simulink library "myLibrary"  (R2023b)
settings: Solver=VariableStepAuto  StartTime=0.0  StopTime=10.0  RelTol=1e-3
undefined symbols (not defined in the file): Cac_n1, ctrl1, Da, Discrete, dtha, ee_sli_rtmsupport, FA, gcbh, Ha, Ini, init_DCline, init_IPC, init_line, init_load, init_SG, init_shunt, init_TH, init_trafo, init_VSC, initMachineBlocks, Ka, Lf, Llkd_pu, Llkq1_pu, magnitude, NET, P, plots_step, q0, Rac_n1, Radd, Rkd_pu, Rkq1_pu, Rload_add, sim_config, sps_rtmsupport, spsSteamTurbineModel, T_DC_NET, T_global, T_IPC, T_load, T_NET, T_SG, T_shunt, T_STATCOM, T_TH, T_trafo, T_VSC, Ts, tstep, Udiff_a, V1
libraries: spsSeriesRLCBranchLib x105, eeGeneralControl x72, $bdroot x70, spsCurrentMeasurementLib x48, spsParallelRLCBranchLib x39, spsVoltageMeasurementLib x33, spsControlledVoltageSourceLib x27, spsFirstOrderFilterLib x16, dspsigops x6, spsThreePhaseVIMeasurementLib x5, spsPLL3phLib x4, spsThreePhaseBreakerLib x3
(part 4 of 12)

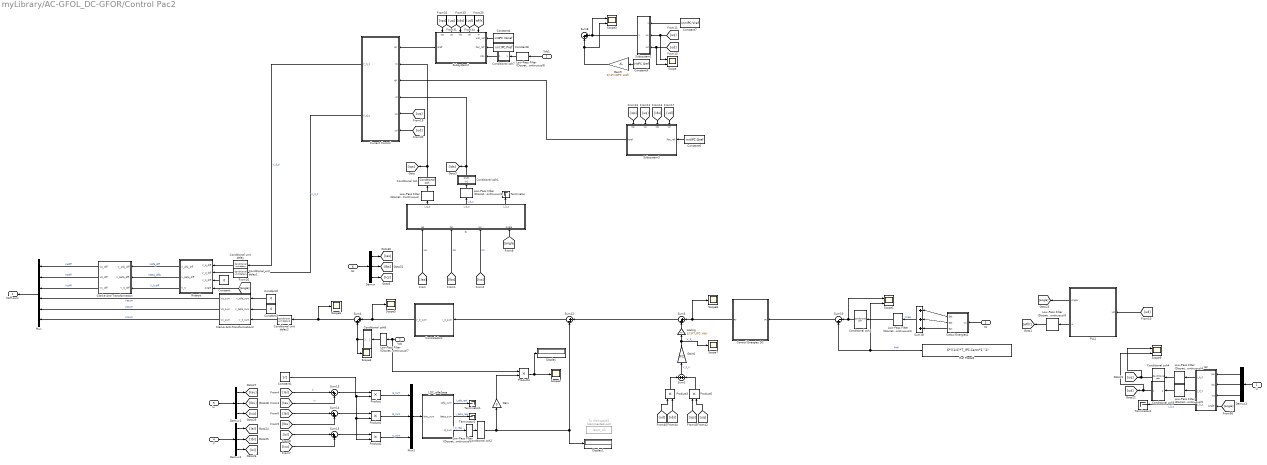
== system myLibrary/AC-GFOL_DC-GFOR/Control Pac2 ==
  U : Inport
  Vdc : Inport  Port=2
  Vs : Inport  Port=3
  Il : Inport  Port=4
  Iu : Inport  Port=5
  Iss : Inport  Port=6
  Calcul Energies2 : Subsystem
  Clarke Anti-Transformation : Subsystem
  Clarke Anti-Transformation2 : Subsystem
  Conditional unit delay : $bdroot/GFOL/Control/Conditional unit delay  SystemSampleTime=-1  VariantActivationTime=update diagram  AllowFlexibleInterface=on  Latency=0  AutoFrameSizeCalculation=off
      link override Constant4: Value=T_IPC.tau_cmd
      link override Unit Delay2: InitialCondition=initIPC.vdiffq  SampleTime=T_IPC.tau_cmd
  Conditional unit delay1 : $bdroot/AC-GFOL_DC-GFOL/Control Pac2/Conditional unit delay1  SystemSampleTime=-1  VariantActivationTime=update diagram  AllowFlexibleInterface=on  Latency=0  AutoFrameSizeCalculation=off
  Conditional unit delay2 : $bdroot/AC-GFOL_DC-GFOL/Control Pac2/Conditional unit delay2  SystemSampleTime=-1  VariantActivationTime=update diagram  AllowFlexibleInterface=on  Latency=0  AutoFrameSizeCalculation=off
  Conditional zoh{,2..4} (4 alike) : $bdroot/AC-GFOL_DC-GFOL/Control Pac2/Conditional zoh  SystemSampleTime=-1  VariantActivationTime=update diagram  AllowFlexibleInterface=on  Latency=0  AutoFrameSizeCalculation=off
  Conditional zoh1 : Subsystem
  Conditional zoh5 : Subsystem
  Conditional zoh7 : Subsystem
  Conditional zoh8 : Subsystem
  Constant : Constant  Value=0
  Constant1 : Constant  Value=1/2
  Constant2 : Constant  Value=0
  Constant3 : Constant  Value=0
  Constant4 : Constant  Value=initIPC.Vdcref
  Constant6 : Constant  Value=initIPC.Qref
  Constant7 : Constant  Value=initIPC.Vref
  Constant8 : Constant  Value=initIPC.Pref
  Constant9 : Constant  Value=initIPC.Qref
  Control Energies DC : Subsystem
  Controladors : Subsystem
  Current Control : Subsystem
  Demux{,1..3} (4 alike) : Demux  Outputs=3
  Display : Display
  Display1 : Display
  Gain : Gain  Gain=3
  Gain6 : Gain  Gain=3/2
  Gain9 : Gain  Gain=2/(3*initIPC.Vref)
  Is : Subsystem
  Is2 : Subsystem
  Low-Pass Filter (Discrete or Continuous) : eeGeneralControl/Low-Pass Filter (Discrete or Continuous)  K=1  T=T_IPC.delay  B=inf  A=-inf  init_option=Specify as parameter  x0=initIPC.idiffq  Ts=0
  Low-Pass Filter (Discrete or Continuous)1 : eeGeneralControl/Low-Pass Filter (Discrete or Continuous)  K=1  T=T_IPC.delay  B=inf  A=-inf  init_option=Specify as parameter  x0=initIPC.idiffd  Ts=0
  Low-Pass Filter (Discrete or Continuous)3 : eeGeneralControl/Low-Pass Filter (Discrete or Continuous)  K=1  T=T_IPC.delay  B=inf  A=-inf  init_option=Specify as parameter  x0=6*((1/2)*T_IPC.Carm*1^2)  Ts=0
  Low-Pass Filter (Discrete or Continuous)4 : eeGeneralControl/Low-Pass Filter (Discrete or Continuous)  K=1  T=T_IPC.delay  B=inf  A=-inf  init_option=Specify as parameter  x0=initIPC.uq  Ts=0
  Low-Pass Filter (Discrete or Continuous)5 : eeGeneralControl/Low-Pass Filter (Discrete or Continuous)  K=1  T=T_IPC.delay  B=inf  A=-inf  init_option=Specify as parameter  x0=initIPC.ud  Ts=0
  Low-Pass Filter (Discrete or Continuous)6 : eeGeneralControl/Low-Pass Filter (Discrete or Continuous)  K=1  T=T_IPC.delay  B=inf  A=-inf  init_option=Specify as parameter  x0=initIPC.isum0_DC  Ts=0
  Low-Pass Filter (Discrete or Continuous)7 : eeGeneralControl/Low-Pass Filter (Discrete or Continuous)  K=1  T=T_IPC.delay  B=inf  A=-inf  init_option=Specify as parameter  x0=initIPC.Vdc  Ts=0
  Low-Pass Filter (Discrete or Continuous)8 : eeGeneralControl/Low-Pass Filter (Discrete or Continuous)  K=1  T=T_IPC.delay  B=inf  A=-inf  init_option=Specify as parameter  x0=initIPC.Vdc  Ts=0
  Low-Pass Filter (Discrete or Continuous)9 : eeGeneralControl/Low-Pass Filter (Discrete or Continuous)  K=1  T=T_IPC.tw  B=inf  A=-inf  init_option=Specify as parameter  x0=2*pi*T_IPC.fb  Ts=0
  Mux : Mux  Inputs=6
  Mux2 : Mux  Inputs=3
  PLL1 : Subsystem
  Product{,1..5} (6 alike) : Product
  Ref Ptotal2 : Constant  Value=6*((1/2)*T_IPC.Carm*1^2)
  Rotació : Subsystem
  Scope{,1,3,9} (4 alike) : Scope  NumInputPorts=2
  Scope{2,4..8} (6 alike) : Scope
  Subsystem1 : Subsystem
      settings: PortSchema="{\"entries\":[{\"content\":{\"sides\":[{\"content\":{\"connectorIds\":[\"Out1\"]},\"type\":\"ConnectorPlacement.EquallySpacedRectSide\",\"uuid\":\"effe47ce-951a-4fb1-8fc1-e963775b8c82\"},{\"content\":{\"connectorIds\":[\"In1\",\"In2\",\"In3\"],\"side\":\"RIGHT\"},\"type\":\"ConnectorPlacement.EquallySpacedRectSide\",\"uuid\":\"a859b59d-6664-4e67-878a-4ecbefd8f8f0\"},{\"content\":{\"connectorIds\":[],\"side\":\"TOP\"},\"type\":\"ConnectorPlacement.EquallySpacedRectSide\",\"uuid\":\"0b762440-c8d9-40a7-a5db-13c46bc0406e\"}]},\"type\":\"ConnectorPlacement.EquallySpacedConnector\",\"uuid\":\"dbc4fef9-6b40-4568-97c6-19f27935f422\"}],\"packageUris\":[\"http://schema.mathworks.com/mf0/Connector/R2020b\"],\"version\":\"1.0\"}"
  Subsystem2 : Subsystem
      settings: PortSchema="{\"entries\":[{\"content\":{\"sides\":[{\"content\":{\"connectorIds\":[\"Out1\"]},\"type\":\"ConnectorPlacement.EquallySpacedRectSide\",\"uuid\":\"dea8424c-00e8-4bd8-a696-176e9d81b4b0\"},{\"content\":{\"connectorIds\":[\"In6\",\"In7\",\"In8\"],\"side\":\"RIGHT\"},\"type\":\"ConnectorPlacement.EquallySpacedRectSide\",\"uuid\":\"15b830a2-0897-480b-96a6-ff349e082a47\"},{\"content\":{\"connectorIds\":[\"In1\",\"In2\",\"In3\",\"In4\",\"In5\"],\"side\":\"TOP\"},\"type\":\"ConnectorPlacement.EquallySpacedRectSide\",\"uuid\":\"07916eec-e3fd-4ba3-9129-5b3a9aa06051\"}]},\"type\":\"ConnectorPlacement.EquallySpacedConnector\",\"uuid\":\"22000632-3c2a-414c-a4d7-471046f1c1a1\"}],\"packageUris\":[\"http://schema.mathworks.com/mf0/Connector/R2020b\"],\"version\":\"1.0\"}"
  Subsystem3 : Subsystem  AncestorBlock=myLibrary/AC-GFOL_DC-GFOR/Control Pac2/Subsystem2
      settings: PortSchema="{\"entries\":[{\"content\":{\"sides\":[{\"content\":{\"connectorIds\":[\"Out1\"]},\"type\":\"ConnectorPlacement.EquallySpacedRectSide\",\"uuid\":\"dea8424c-00e8-4bd8-a696-176e9d81b4b0\"},{\"content\":{\"connectorIds\":[\"In5\"],\"side\":\"RIGHT\"},\"type\":\"ConnectorPlacement.EquallySpacedRectSide\",\"uuid\":\"15b830a2-0897-480b-96a6-ff349e082a47\"},{\"content\":{\"connectorIds\":[\"In1\",\"In2\",\"In3\",\"In4\"],\"side\":\"TOP\"},\"type\":\"ConnectorPlacement.EquallySpacedRectSide\",\"uuid\":\"07916eec-e3fd-4ba3-9129-5b3a9aa06051\"}]},\"type\":\"ConnectorPlacement.EquallySpacedConnector\",\"uuid\":\"22000632-3c2a-414c-a4d7-471046f1c1a1\"}],\"packageUris\":[\"http://schema.mathworks.com/mf0/Connector/R2020b\"],\"version\":\"1.0\"}"
  Sum1 : Sum
  Sum12 : Sum  Inputs=|+-
  Sum{3..4,8,13..15} (6 alike) : Sum  Inputs=|++
  Sum18 : Sum  Inputs=|+++
  Sum19 : Sum  Inputs=|-+
  Terminator{,1..2,4} (4 alike) : Terminator
  To Workspace2 : ToWorkspace  Commented=on  VariableName=isum_n1  SampleTime=plots_step
  Vdc1 : InportShadow  Port=2
  l_DC_alfa/beta : Subsystem
  scaling : Gain  Gain=1/(3*T_IPC.Vdc)
  Vdiff-sum : Outport
  wires:
  Low-Pass Filter (Discrete or Continuous)9/1 -> [wfilt]
  PLL1/2(w) -> Low-Pass Filter (Discrete or Continuous)9/1
  Is/3(I_0_s) -> Terminator/1
  Low-Pass Filter (Discrete or Continuous)7/1 -> Conditional zoh8/1(In1)
  Low-Pass Filter (Discrete or Continuous)3/1 -> Conditional zoh3/1
  Low-Pass Filter (Discrete or Continuous)4/1 -> Conditional zoh4/1
  Low-Pass Filter (Discrete or Continuous)5/1 -> Conditional zoh5/1(In1)
  Low-Pass Filter (Discrete or Continuous)1/1 -> Conditional zoh1/1(In1)
  Low-Pass Filter (Discrete or Continuous)/1 -> Conditional zoh/1
  Ref Ptotal2/1 -> Scope1/2, Sum19/2  "Pref"
  Calcul Energies2/1(Eat) -> Sum18/1
  Constant2/1 -> Clarke Anti-Transformation2/1(V_alfa_sum)
  Constant3/1 -> Clarke Anti-Transformation2/2(V_beta_sum)
  Mux/1 -> Vdiff-sum/1
  Clarke Anti-Transformation2/1(Va_sum) -> Mux/4  "Vasum"
  Clarke Anti-Transformation2/2(Vb_sum) -> Mux/5  "Vbsum"
  Clarke Anti-Transformation/3(Vc_diff) -> Mux/3  "Vcdiff"
  Clarke Anti-Transformation/2(Vb_diff) -> Mux/2  "Vbdiff"
  Clarke Anti-Transformation/1(Va_diff) -> Mux/1  "Vadiff"
  Rotació/1(V_alfa_diff) -> Clarke Anti-Transformation/1(V_alfa_diff)  "Valfa_diff"
  Rotació/3(V_0) -> Clarke Anti-Transformation/3(V_0_diff)  "V_0_diff"
  [Ias] -> Is/1(Ias)  "Ias"
  [Ics] -> Is/3(Ics)  "Ics"
  [Ibs] -> Is/2(Ibs)  "Ibs"
  Rotació/2(V_beta_diff) -> Clarke Anti-Transformation/2(V_beta_dfff)  "Vbeta_diffa"
  Mux2/1 -> l_DC_alfa/beta/1(Iabc_sum)
  Product/1 -> Mux2/1  "Ia_sum"
  [Ial] -> Sum13/1  "Il"
  [Iau] -> Sum13/2  "Iu"
  Sum13/1 -> Product/1
  Constant1/1 -> Product2/2, Product1/2, Product/2
  Product1/1 -> Mux2/2  "Ib_sum"
  [Ibl] -> Sum14/1
  [Ibu] -> Sum14/2
  Sum14/1 -> Product1/1
  Product2/1 -> Mux2/3  "Ic_sum"
  [Icl] -> Sum15/1
  [Icu] -> Sum15/2
  Sum15/1 -> Product2/1
  Clarke Anti-Transformation2/3(Vc_sum) -> Mux/6  "Vcsum"
  Iu/1 -> Demux1/1
  Demux2/2 -> [Ibl]
  Demux1/1 -> [Iau]
  Demux1/3 -> [Icu]
  Il/1 -> Demux2/1
  Demux2/3 -> [Icl]
  Demux2/1 -> [Ial]
  Demux1/2 -> [Ibu]
  Demux3/2 -> Is2/2(Ibs)
  [angle] -> Is2/4(Angle)
  PLL1/1(Angle) -> [angle]
  [ud] -> PLL1/1(Ud)
  U/1 -> Demux3/1
  Demux3/3 -> Is2/3(Ics)
  Demux3/1 -> Is2/1(Ias)
  Demux/1 -> [Ias]
  Demux/2 -> [Ibs]
  Demux/3 -> [Ics]
  Iss/1 -> Demux/1
  Vs/1 -> Calcul Energies2/1(Vs)
  Calcul Energies2/3(Ect) -> Sum18/3
  Calcul Energies2/2(Ebt) -> Sum18/2
  [angle] -> Is/4(Angle)
  [angle] -> Rotació/4(Angle)
  Current Control/1(V_q_s) -> Conditional unit delay/1  "V_0_s"
  [uq] -> Current Control/5(uq)
  [ud] -> Current Control/6(ud)
  Controladors/1(V_0_sum) -> Scope5/1, Sum4/1
  Sum12/1 -> Controladors/1(I_0_sum)
  Sum19/1 -> Control Energies DC/1(Pt)
  Constant7/1 -> Subsystem1/1(uref)
  [uq] -> Scope/1, Subsystem1/2(uq)
  [ud] -> Scope/2, Subsystem1/3(ud)
  Sum4/1 -> Scope6/1, Conditional unit delay2/1
  Is2/3(I_0_s) -> Terminator4/1  "I_0_s"
  Subsystem2/1(iqref) -> Current Control/1(Iq*)
  [ud] -> Product3/1
  [uq] -> Product5/2
  Gain6/1 -> Scope7/1, scaling/1  "V_0_"
  Sum1/1 -> Gain6/1  "V_0_s"
  Product5/1 -> Sum1/2
  Control Energies DC/1(Pt') -> Scope8/1, Sum3/1
  [iqs] -> Product5/1
  scaling/1 -> Sum3/2
  Sum3/1 -> Sum12/1
  Product3/1 -> Sum1/1
  [ids] -> Product3/2
  Subsystem1/1(idref) -> Scope3/1, Sum8/1
  Constant9/1 -> Gain9/1
  Gain9/1 -> Scope3/2, Sum8/2
  Current Control/2(V_d_s) -> Conditional unit delay1/1  "V_0_s"
  Constant/1 -> Rotació/3(V_0_diff)
  l_DC_alfa/beta/1(Ialfa_sum) -> Terminator1/1  "I_afa_real"
  l_DC_alfa/beta/2(Ibeta_sum) -> Terminator2/1  "I_beta_real"
  Constant8/1 -> Subsystem2/7(Pac_ref)
  Vdc1/1 -> Low-Pass Filter (Discrete or Continuous)8/1
  Low-Pass Filter (Discrete or Continuous)8/1 -> Conditional zoh7/1(In1)
  Constant4/1 -> Subsystem2/6(Vdc_ref)
  [wfilt] -> Subsystem2/5(w)
  [ud] -> Subsystem2/4(ud)
  [ids] -> Subsystem2/3(ids)
  [uq] -> Subsystem2/2(uq)
  [iqs] -> Subsystem2/1(iqs)
  Gain/1 -> Product4/2
  Product4/1 -> Display/1, Scope2/1
  [uq] -> Subsystem3/2(uq)
  [ud] -> Subsystem3/4(ud)
  [ids] -> Subsystem3/3(ids)
  Constant6/1 -> Subsystem3/5(Pac_ref)
  [iqs] -> Subsystem3/1(iqs)
  Subsystem3/1(iqref) -> Current Control/3(Id*)
  Conditional unit delay1/1 -> Rotació/2(V_d_diff)
  Conditional unit delay/1 -> Rotació/1(V_q_diff)
  Vdc/1 -> Low-Pass Filter (Discrete or Continuous)7/1, Product4/1
  Conditional unit delay2/1 -> Clarke Anti-Transformation2/3(V_0_sum)
  Conditional zoh7/1(Out1) -> Subsystem2/8(Vdc)
  Conditional zoh8/1(Out1) -> Scope4/1, Sum4/2
  l_DC_alfa/beta/3(I0_sum) -> Low-Pass Filter (Discrete or Continuous)6/1  "I_0_real"
  Low-Pass Filter (Discrete or Continuous)6/1 -> Conditional zoh2/1
  Conditional zoh2/1 -> Gain/1, Sum12/2, Display1/1
  Sum18/1 -> Low-Pass Filter (Discrete or Continuous)3/1  "Preal"
  Conditional zoh3/1 -> Scope1/1, Sum19/1
  Is2/1(I_q_s) -> Low-Pass Filter (Discrete or Continuous)4/1
  Is2/2(I_d_s) -> Low-Pass Filter (Discrete or Continuous)5/1
  Conditional zoh5/1(Out1) -> Scope9/2, [ud]
  Conditional zoh4/1 -> Scope9/1, [uq]
  Is/1(I_q_s) -> Low-Pass Filter (Discrete or Continuous)/1
  Conditional zoh/1 -> Current Control/2(Iq), [iqs]
  Is/2(I_d_s) -> Low-Pass Filter (Discrete or Continuous)1/1  "I_d_s"
  Conditional zoh1/1(Out1) -> Current Control/4(Id), [ids]

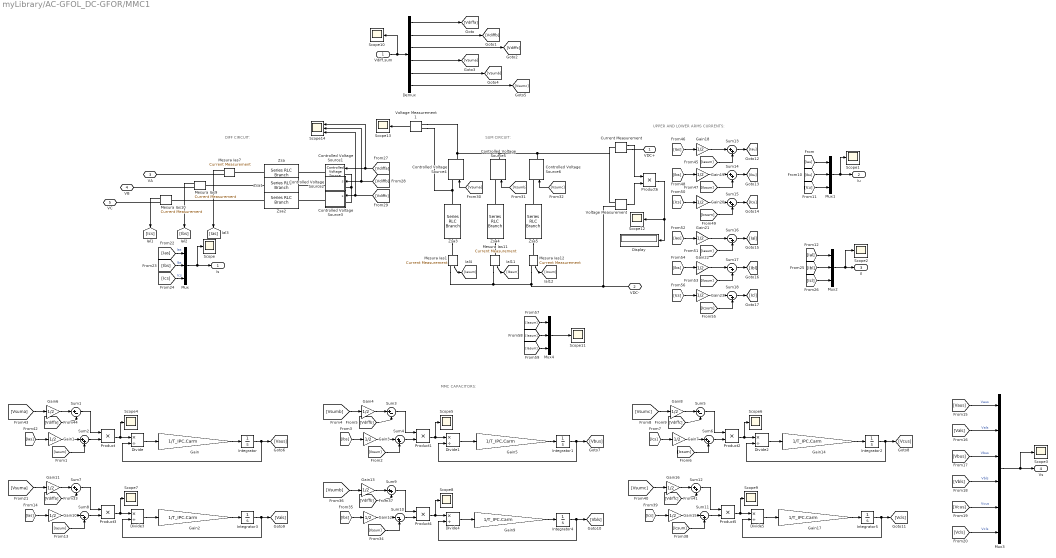
== system myLibrary/AC-GFOL_DC-GFOR/MMC1 ==
  note: DIFF CIRCUIT:
  note: SUM CIRCUIT:
  note: MMC CAPACITORS:
  note: UPPER AND LOWER ARMS CURRENTS:
  Vdiff,sum : Inport
  Controlled Voltage Source1 : spsControlledVoltageSourceLib/Controlled Voltage Source  Initialize=on  Source_Type=AC  Amplitude=initIPC.Udiff_mag  Phase=initIPC.angle_vdiff  Frequency=T_IPC.fb  Measurements=None
  Controlled Voltage Source2 : Subsystem  DialogController=POWERSYS.PowerSysDialog  LoadFcn=sps_rtmsupport('LoadFcn',gcbh);  StartFcn=sps_rtmsupport('StartFcn',gcbh);  StopFcn=sps_rtmsupport('StopFcn',gcbh);  mask(Controlled Voltage Source){Initialize=on, Source_Type=AC, Amplitude=initIPC.Udiff_mag, Phase=initIPC.angle_vdiff-120, Frequency=T_IPC.fb, Measurements=None}
      mask prompts: Source_Type "Source type"; Amplitude "Initial amplitude (V):"; Phase "Initial phase (deg):"; Frequency "Initial frequency (Hz):"
      mask help:
      | Converts the Simulink input signal into an equivalent voltage source. The generated voltage is driven by the input signal of the block.
      |
      | You can initialize your circuit with a specific AC or DC voltage. If you want to start the simulation in steady-state, the block input must be connected to a signal starting as a sinusoidal or DC waveform corresponding to the initial values.
      mask init:
      | powericon('psbloadfunction',gcb,'goto','Initialize');
      | powericon('ControlledSourcesCback',gcb);
      | power_initmask();
      settings: LibrarySourceBlock=spsControlledVoltageSourceLib/Controlled Voltage Source  CopyFcn=sps_rtmsupport('CopyFcn',gcbh); powericon('psbloadfunction',gcb,'goto','UpdateGotoTag');  DeleteFcn=sps_rtmsupport('DeleteFcn',gcbh);  UndoDeleteFcn=sps_rtmsupport('UndoDeleteFcn',gcbh);  ModelCloseFcn=sps_rtmsupport('ModelCloseFcn',gcbh);  PreSaveFcn=sps_rtmsupport('PreSaveFcn',gcbh);  PostSaveFcn=sps_rtmsupport('PostSaveFcn',gcbh);  NameChangeFcn=sps_rtmsupport('NameChangeFcn',gcbh);  PreCopyFcn=sps_rtmsupport('PreCopyFcn',gcbh);  OpenFcn=sps_rtmsupport('OpenFcn',gcbh, [1 2 6]);  CloseFcn=sps_rtmsupport('CloseFcn',gcbh);  PreDeleteFcn=sps_rtmsupport('PreDeleteFcn',gcbh);
      mask Help: helpview(psbhelp);
      mask Callback Initialize: powericon('ControlledSourcesCback',gcb);
      mask TypeOptions Source_Type: AC | DC
      mask Callback Source_Type: powericon('ControlledSourcesCback',gcb);
      mask TypeOptions Measurements: None | Voltage
      mask Display: plot(-50,-35,50,50-15,[0,9,18,24,29,30,29,24,18,9,0,-9,-18,-24,-29,-30,-29,-24,-18,-9,0],[30,29,24,18,9,0,-9,-18,-24,-29,-30,-29,-24,-18,-9,0,9,18,24,29,30],[0,9,18,24,29,30,29,24,18,9,0,-9,-18,-24,-29,-30,-29,-24,-18,-9,0]./-2.4,[1 2 3 4 5 6 7 8 9 10 11 12 13 14 15 16 17 18 19 20 21].*1.5-15);
  Controlled Voltage Source3 : Subsystem  DialogController=POWERSYS.PowerSysDialog  LoadFcn=sps_rtmsupport('LoadFcn',gcbh);  StartFcn=sps_rtmsupport('StartFcn',gcbh);  StopFcn=sps_rtmsupport('StopFcn',gcbh);  mask(Controlled Voltage Source){Initialize=on, Source_Type=AC, Amplitude=initIPC.Udiff_mag, Phase=initIPC.angle_vdiff+120, Frequency=T_IPC.fb, Measurements=None}
      mask prompts: Source_Type "Source type"; Amplitude "Initial amplitude (V):"; Phase "Initial phase (deg):"; Frequency "Initial frequency (Hz):"
      mask help:
      | Converts the Simulink input signal into an equivalent voltage source. The generated voltage is driven by the input signal of the block.
      |
      | You can initialize your circuit with a specific AC or DC voltage. If you want to start the simulation in steady-state, the block input must be connected to a signal starting as a sinusoidal or DC waveform corresponding to the initial values.
      mask init:
      | powericon('psbloadfunction',gcb,'goto','Initialize');
      | powericon('ControlledSourcesCback',gcb);
      | power_initmask();
      settings: LibrarySourceBlock=spsControlledVoltageSourceLib/Controlled Voltage Source  CopyFcn=sps_rtmsupport('CopyFcn',gcbh); powericon('psbloadfunction',gcb,'goto','UpdateGotoTag');  DeleteFcn=sps_rtmsupport('DeleteFcn',gcbh);  UndoDeleteFcn=sps_rtmsupport('UndoDeleteFcn',gcbh);  ModelCloseFcn=sps_rtmsupport('ModelCloseFcn',gcbh);  PreSaveFcn=sps_rtmsupport('PreSaveFcn',gcbh);  PostSaveFcn=sps_rtmsupport('PostSaveFcn',gcbh);  NameChangeFcn=sps_rtmsupport('NameChangeFcn',gcbh);  PreCopyFcn=sps_rtmsupport('PreCopyFcn',gcbh);  OpenFcn=sps_rtmsupport('OpenFcn',gcbh, [1 2 6]);  CloseFcn=sps_rtmsupport('CloseFcn',gcbh);  PreDeleteFcn=sps_rtmsupport('PreDeleteFcn',gcbh);
      mask Help: helpview(psbhelp);
      mask Callback Initialize: powericon('ControlledSourcesCback',gcb);
      mask TypeOptions Source_Type: AC | DC
      mask Callback Source_Type: powericon('ControlledSourcesCback',gcb);
      mask TypeOptions Measurements: None | Voltage
      mask Display: plot(-50,-35,50,50-15,[0,9,18,24,29,30,29,24,18,9,0,-9,-18,-24,-29,-30,-29,-24,-18,-9,0],[30,29,24,18,9,0,-9,-18,-24,-29,-30,-29,-24,-18,-9,0,9,18,24,29,30],[0,9,18,24,29,30,29,24,18,9,0,-9,-18,-24,-29,-30,-29,-24,-18,-9,0]./-2.4,[1 2 3 4 5 6 7 8 9 10 11 12 13 14 15 16 17 18 19 20 21].*1.5-15);
  Controlled Voltage Source4 : spsControlledVoltageSourceLib/Controlled Voltage Source  Initialize=on  Source_Type=DC  Amplitude=initIPC.Usuma  Phase=0  Frequency=0  Measurements=None
  Controlled Voltage Source5 : spsControlledVoltageSourceLib/Controlled Voltage Source  Initialize=on  Source_Type=DC  Amplitude=initIPC.Usumb  Phase=angle(Udiff_a)*180/pi  Frequency=60  Measurements=None
  Controlled Voltage Source6 : spsControlledVoltageSourceLib/Controlled Voltage Source  Initialize=on  Source_Type=DC  Amplitude=initIPC.Usumc  Phase=angle(Udiff_a)*180/pi  Frequency=60  Measurements=None
  Current Measurement : spsCurrentMeasurementLib/Current Measurement  PhasorSimulation=off  OutputType=Complex  PSBequivalent=0
  Demux : Demux  Outputs=6
  Display : Display
  Divide{,1..5} (6 alike) : Product  Inputs=*/
  Gain{,2,5,9,14,17} (6 alike) : Gain  Gain=1/T_IPC.Carm
  Gain{1,3..4,6..8,10..13,15..16,18..23} (18 alike) : Gain  Gain=1/2
  Integrator{,1..5} (6 alike) : Integrator  InitialCondition=1
  Mesura Ias{1,7,9..12} (6 alike) : spsCurrentMeasurementLib/Current Measurement  PhasorSimulation=off  OutputType=Complex  PSBequivalent=0
  Mux{,1..2,4} (4 alike) : Mux  Inputs=3
  Mux3 : Mux  Inputs=6
  Product{,1..6} (7 alike) : Product
  Scope{,1..13} (14 alike) : Scope
  Scope14 : Scope  NumInputPorts=3
  Sum1 : Sum  Inputs=|+-
  Sum{8,10..11,16..18} (6 alike) : Sum  Inputs=|-+
  Sum{2,4,6..7,9,12..15} (9 alike) : Sum  Inputs=|++
  Sum3 : Sum  Inputs=|+-
  Sum5 : Sum  Inputs=|+-
  Voltage Measurement : spsVoltageMeasurementLib/Voltage Measurement  PhasorSimulation=off  OutputType=Complex  PSBequivalent=0
  Voltage Measurement1 : spsVoltageMeasurementLib/Voltage Measurement  PhasorSimulation=off  OutputType=Complex  PSBequivalent=0
  Zsa : spsSeriesRLCBranchLib/Series RLC Branch  LConnTagsString=__new0  RConnTagsString=__new0  BranchType=RL  Resistance=T_IPC.Rc+T_IPC.Ra/2  Inductance=T_IPC.Lc+T_IPC.La/2  SetiL0=on  InitialCurrent=initIPC.Isa  Capacitance=1e-6  Setx0=off  InitialVoltage=0  Measurements=None
  Zsa1 : spsSeriesRLCBranchLib/Series RLC Branch  LConnTagsString=__new0  RConnTagsString=__new0  BranchType=RL  Resistance=T_IPC.Rc+T_IPC.Ra/2  Inductance=T_IPC.Lc+T_IPC.La/2  SetiL0=on  InitialCurrent=initIPC.Isb  Capacitance=1e-6  Setx0=off  InitialVoltage=0  Measurements=None
  Zsa2 : spsSeriesRLCBranchLib/Series RLC Branch  LConnTagsString=__new0  RConnTagsString=__new0  BranchType=RL  Resistance=T_IPC.Rc+T_IPC.Ra/2  Inductance=T_IPC.Lc+T_IPC.La/2  SetiL0=on  InitialCurrent=initIPC.Isc  Capacitance=1e-6  Setx0=off  InitialVoltage=0  Measurements=None
  Zsa3 : spsSeriesRLCBranchLib/Series RLC Branch  LConnTagsString=__new0  RConnTagsString=__new0  BranchType=RL  Resistance=2*T_IPC.Ra  Inductance=2*T_IPC.La  SetiL0=on  InitialCurrent=initIPC.isum0_DC  Capacitance=1e-6  Setx0=off  InitialVoltage=0  Measurements=None
  Zsa4 : spsSeriesRLCBranchLib/Series RLC Branch  LConnTagsString=__new0  RConnTagsString=__new0  BranchType=RL  Resistance=2*T_IPC.Ra  Inductance=2*T_IPC.La  SetiL0=on  InitialCurrent=initIPC.isum0_DC  Capacitance=1e-6  Setx0=off  InitialVoltage=0  Measurements=None
  Zsa5 : spsSeriesRLCBranchLib/Series RLC Branch  LConnTagsString=__new0  RConnTagsString=__new0  BranchType=RL  Resistance=2*T_IPC.Ra  Inductance=2*T_IPC.La  SetiL0=on  InitialCurrent=initIPC.isum0_DC  Capacitance=1e-6  Setx0=off  InitialVoltage=0  Measurements=None
  VDC+ : PMIOPort  Side=Right
  VDC- : PMIOPort  Port=2  Side=Right
  VA : PMIOPort  Port=3  Side=Left
  VB : PMIOPort  Port=4  Side=Left
  VC : PMIOPort  Port=5  Side=Left
  Is : Outport
  Iu : Outport  Port=2
  Il : Outport  Port=3
  Vs : Outport  Port=4
  wires:
  Mux4/1 -> Scope11/1
  [Iasum] -> Mux4/3
  [Iasum] -> Mux4/2
  [Iasum] -> Mux4/1
  Mesura Ias10/1 -> [Ics]
  Mesura Ias7/1 -> [Ias]
  Mesura Ias9/1 -> [Ibs]
  Vdiff,sum/1 -> Demux/1, Scope10/1
  Demux/5 -> [Vsumb]
  Demux/6 -> [Vsumc]
  Demux/1 -> [Vdiffa]
  Demux/3 -> [Vdiffc]
  Demux/2 -> [Vdiffb]
  Demux/4 -> [Vsuma]
  Mux/1 -> Scope/1, Is/1
  [Ics] -> Mux/3  "Ics"
  [Ibs] -> Mux/2  "Ibs"
  [Ias] -> Mux/1  "Ias"
  [Iau] -> Mux1/1
  [Ibu] -> Mux1/2
  [Icu] -> Mux1/3
  Mux1/1 -> Scope1/1, Iu/1
  [Ial] -> Mux2/1
  Mux2/1 -> Scope2/1, Il/1
  [Icl] -> Mux2/3
  [Vaus] -> Mux3/1  "Vaus"
  [Vals] -> Mux3/2  "Vals"
  [Vbus] -> Mux3/3  "Vbus"
  [Vbls] -> Mux3/4  "Vbls"
  [Vcus] -> Mux3/5  "Vcus"
  [Vcls] -> Mux3/6  "Vcls"
  Mux3/1 -> Scope3/1, Vs/1
  Sum2/1 -> Product/2
  Product/1 -> Scope4/1, Divide/1
  Divide/1 -> Gain/1
  Gain/1 -> Integrator/1
  Integrator/1 -> [Vaus], Divide/2
  [Vdiffa] -> Scope14/1, Controlled Voltage Source1/1
  [Vdiffb] -> Scope14/2, Controlled Voltage Source2/1(s)
  Mesura Ias1/1 -> [Iasum]
  Mesura Ias11/1 -> [Ibsum]
  Mesura Ias12/1 -> [Icsum]
  [Vsuma] -> Controlled Voltage Source4/1
  [Vsumb] -> Controlled Voltage Source5/1
  [Vsumc] -> Controlled Voltage Source6/1
  Gain6/1 -> Sum1/1
  [Vdiffa] -> Sum1/2
  [Iasum] -> Sum2/2
  Gain1/1 -> Sum2/1
  [Ias] -> Gain1/1
  [Vsuma] -> Gain6/1
  Sum1/1 -> Product/1
  Sum3/1 -> Product1/1
  [Vsumb] -> Gain4/1
  [Ibs] -> Gain3/1
  Gain3/1 -> Sum4/1
  [Ibsum] -> Sum4/2
  [Vdiffb] -> Sum3/2
  Gain4/1 -> Sum3/1
  Integrator1/1 -> Divide1/2, [Vbus]
  Gain5/1 -> Integrator1/1
  Divide1/1 -> Gain5/1
  Product1/1 -> Divide1/1, Scope5/1
  Sum4/1 -> Product1/2
  Sum6/1 -> Product2/2
  Product2/1 -> Scope6/1, Divide2/1
  Divide2/1 -> Gain14/1
  Gain14/1 -> Integrator2/1
  Integrator2/1 -> [Vcus], Divide2/2
  Gain8/1 -> Sum5/1
  [Vdiffc] -> Sum5/2
  [Icsum] -> Sum6/2
  Gain7/1 -> Sum6/1
  [Ics] -> Gain7/1
  [Vsumc] -> Gain8/1
  Sum5/1 -> Product2/1
  Sum7/1 -> Product3/1
  [Vsuma] -> Gain11/1
  [Ias] -> Gain10/1
  Gain10/1 -> Sum8/1
  [Iasum] -> Sum8/2
  [Vdiffa] -> Sum7/2
  Gain11/1 -> Sum7/1
  Integrator3/1 -> Divide3/2, [Vals]
  Gain2/1 -> Integrator3/1
  Divide3/1 -> Gain2/1
  Product3/1 -> Divide3/1, Scope7/1
  Sum8/1 -> Product3/2
  Sum10/1 -> Product4/2
  Product4/1 -> Scope8/1, Divide4/1
  Divide4/1 -> Gain9/1
  Gain9/1 -> Integrator4/1
  Integrator4/1 -> [Vbls], Divide4/2
  Gain13/1 -> Sum9/1
  [Vdiffb] -> Sum9/2
  [Ibsum] -> Sum10/2
  Gain12/1 -> Sum10/1
  [Ibs] -> Gain12/1
  [Vsumb] -> Gain13/1
  Sum9/1 -> Product4/1
  Sum12/1 -> Product5/1
  [Vsumc] -> Gain16/1
  [Ics] -> Gain15/1
  Gain15/1 -> Sum11/1
  [Icsum] -> Sum11/2
  [Vdiffc] -> Sum12/2
  Gain16/1 -> Sum12/1
  Integrator5/1 -> Divide5/2, [Vcls]
  Gain17/1 -> Integrator5/1
  Divide5/1 -> Gain17/1
  Product5/1 -> Divide5/1, Scope9/1
  Sum11/1 -> Product5/2
  [Ias] -> Gain18/1
  Gain18/1 -> Sum13/1
  [Iasum] -> Sum13/2
  Sum13/1 -> [Iau]
  Sum14/1 -> [Ibu]
  [Ibsum] -> Sum14/2
  Gain19/1 -> Sum14/1
  [Ibs] -> Gain19/1
  [Ics] -> Gain20/1
  Gain20/1 -> Sum15/1
  [Icsum] -> Sum15/2
  Sum15/1 -> [Icu]
  [Iasum] -> Sum16/2
  [Ias] -> Gain21/1
  Gain21/1 -> Sum16/1
  Sum16/1 -> [Ial]
  Sum17/1 -> [Ibl]
  Gain22/1 -> Sum17/1
  [Ibs] -> Gain22/1
  [Ibsum] -> Sum17/2
  [Icsum] -> Sum18/2
  [Ics] -> Gain23/1
  Gain23/1 -> Sum18/1
  Sum18/1 -> [Icl]
  [Ibl] -> Mux2/2
  Current Measurement/1 -> Product6/1
  Voltage Measurement/1 -> Product6/2
  Product6/1 -> Display/1, Scope12/1
  Voltage Measurement1/1 -> Scope13/1
  [Vdiffc] -> Controlled Voltage Source3/1(s), Scope14/3
  connections:
  Zsa5/RConn1 -- Mesura Ias12/LConn1
  Zsa5/LConn1 -- Controlled Voltage Source6/LConn1
  Zsa4/RConn1 -- Mesura Ias11/LConn1
  Zsa4/LConn1 -- Controlled Voltage Source5/LConn1
  Zsa3/RConn1 -- Mesura Ias1/LConn1
  Zsa3/LConn1 -- Voltage Measurement1/LConn2 -- Controlled Voltage Source4/LConn1
  Mesura Ias7/RConn1 -- VA/RConn1
  Mesura Ias9/RConn1 -- VB/RConn1
  Mesura Ias10/RConn1 -- VC/RConn1
  Zsa/RConn1 -- Mesura Ias7/LConn1
  Zsa1/RConn1 -- Mesura Ias9/LConn1
  Zsa2/RConn1 -- Mesura Ias10/LConn1
  Controlled Voltage Source1/RConn1 -- Zsa/LConn1
  Controlled Voltage Source2/RConn1 -- Zsa1/LConn1
  Controlled Voltage Source3/RConn1 -- Zsa2/LConn1
  Controlled Voltage Source1/LConn1 -- Controlled Voltage Source3/LConn1 -- Controlled Voltage Source2/LConn1
  Controlled Voltage Source6/RConn1 -- Current Measurement/LConn1 -- Voltage Measurement/LConn1 -- Controlled Voltage Source5/RConn1 -- Voltage Measurement1/LConn1 -- Controlled Voltage Source4/RConn1
  Mesura Ias1/RConn1 -- Mesura Ias11/RConn1 -- Mesura Ias12/RConn1 -- Voltage Measurement/LConn2 -- VDC-/RConn1
  Current Measurement/RConn1 -- VDC+/RConn1

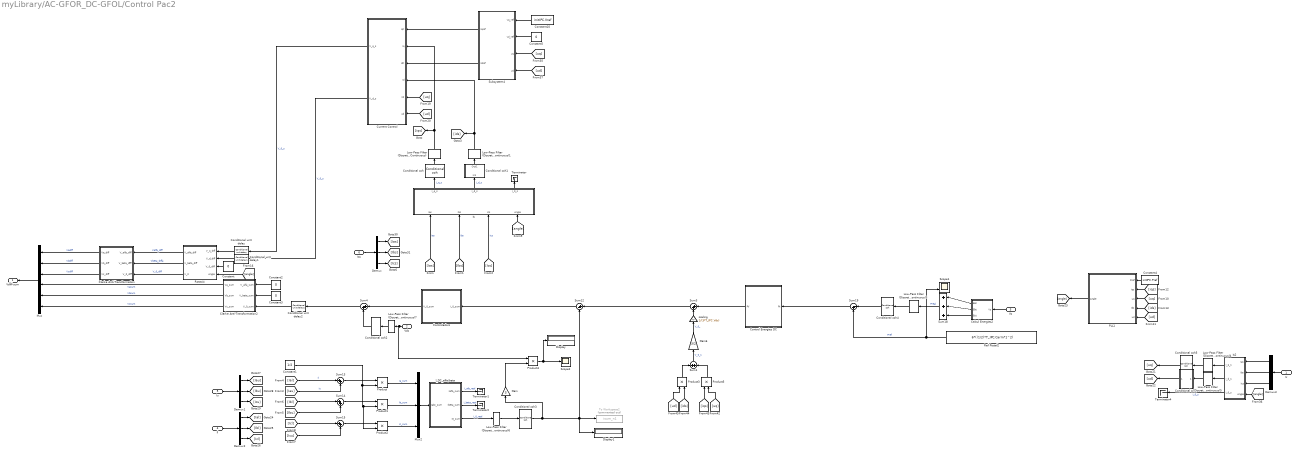
== system myLibrary/AC-GFOR_DC-GFOL/Control Pac2 ==
  U : Inport
  Vdc : Inport  Port=2
  Vs : Inport  Port=3
  Il : Inport  Port=4
  Iu : Inport  Port=5
  Iss : Inport  Port=6
  Calcul Energies2 : Subsystem
  Clarke Anti-Transformation : Subsystem
  Clarke Anti-Transformation2 : Subsystem
  Conditional unit delay : $bdroot/GFOL/Control/Conditional unit delay  SystemSampleTime=-1  VariantActivationTime=update diagram  AllowFlexibleInterface=on  Latency=0  AutoFrameSizeCalculation=off
      link override Constant4: Value=T_IPC.tau_cmd
      link override Unit Delay2: InitialCondition=initIPC.vdiffq  SampleTime=T_IPC.tau_cmd
  Conditional unit delay1 : $bdroot/AC-GFOL_DC-GFOL/Control Pac2/Conditional unit delay1  SystemSampleTime=-1  VariantActivationTime=update diagram  AllowFlexibleInterface=on  Latency=0  AutoFrameSizeCalculation=off
  Conditional unit delay2 : $bdroot/AC-GFOL_DC-GFOL/Control Pac2/Conditional unit delay2  SystemSampleTime=-1  VariantActivationTime=update diagram  AllowFlexibleInterface=on  Latency=0  AutoFrameSizeCalculation=off
  Conditional zoh{,2..5} (5 alike) : $bdroot/AC-GFOL_DC-GFOL/Control Pac2/Conditional zoh  SystemSampleTime=-1  VariantActivationTime=update diagram  AllowFlexibleInterface=on  Latency=0  AutoFrameSizeCalculation=off
  Conditional zoh1 : Subsystem
  Conditional zoh6 : Subsystem
  Constant{,2..3,5} (4 alike) : Constant  Value=0
  Constant1 : Constant  Value=1/2
  Constant10 : Constant  Value=initIPC.Vref
  Constant4 : Constant  Value=initIPC.Pref
  Control Energies DC : Subsystem
  Controladors : Subsystem
  Current Control : Subsystem
  Demux{,1..3} (4 alike) : Demux  Outputs=3
  Display : Display
  Display1 : Display
  Gain : Gain  Gain=3
  Gain6 : Gain  Gain=3/2
  Is : Subsystem
  Is2 : Subsystem
  Low-Pass Filter (Discrete or Continuous) : eeGeneralControl/Low-Pass Filter (Discrete or Continuous)  K=1  T=T_IPC.delay  B=inf  A=-inf  init_option=Specify as parameter  x0=initIPC.idiffq  Ts=0
  Low-Pass Filter (Discrete or Continuous)1 : eeGeneralControl/Low-Pass Filter (Discrete or Continuous)  K=1  T=T_IPC.delay  B=inf  A=-inf  init_option=Specify as parameter  x0=initIPC.idiffd  Ts=0
  Low-Pass Filter (Discrete or Continuous)3 : eeGeneralControl/Low-Pass Filter (Discrete or Continuous)  K=1  T=T_IPC.delay  B=inf  A=-inf  init_option=Specify as parameter  x0=6*((1/2)*T_IPC.Carm*1^2)  Ts=0
  Low-Pass Filter (Discrete or Continuous)4 : eeGeneralControl/Low-Pass Filter (Discrete or Continuous)  K=1  T=T_IPC.delay  B=inf  A=-inf  init_option=Specify as parameter  x0=initIPC.uq  Ts=0
  Low-Pass Filter (Discrete or Continuous)5 : eeGeneralControl/Low-Pass Filter (Discrete or Continuous)  K=1  T=T_IPC.delay  B=inf  A=-inf  init_option=Specify as parameter  x0=initIPC.ud  Ts=0
  Low-Pass Filter (Discrete or Continuous)6 : eeGeneralControl/Low-Pass Filter (Discrete or Continuous)  K=1  T=T_IPC.delay  B=inf  A=-inf  init_option=Specify as parameter  x0=initIPC.isum0_DC  Ts=0
  Low-Pass Filter (Discrete or Continuous)7 : eeGeneralControl/Low-Pass Filter (Discrete or Continuous)  K=1  T=T_IPC.delay  B=inf  A=-inf  init_option=Specify as parameter  x0=initIPC.Vdc  Ts=0
  Mux : Mux  Inputs=6
  Mux2 : Mux  Inputs=3
  PLL1 : Subsystem
  Product{,1..5} (6 alike) : Product
  Ref Ptotal2 : Constant  Value=6*((1/2)*T_IPC.Carm*1^2)
  Rotació : Subsystem
  Scope1 : Scope  NumInputPorts=2
  Scope2 : Scope
  Subsystem4 : Subsystem
  Sum1 : Sum
  Sum12 : Sum  Inputs=|+-
  Sum{3..4,13..15} (5 alike) : Sum  Inputs=|++
  Sum18 : Sum  Inputs=|+++
  Sum19 : Sum  Inputs=|-+
  Terminator{,1..2,4} (4 alike) : Terminator
  To Workspace2 : ToWorkspace  Commented=on  VariableName=isum_n1  SampleTime=plots_step
  l_DC_alfa/beta : Subsystem
  scaling : Gain  Gain=1/(3*T_IPC.Vdc)
  Vdiff-sum : Outport
  wires:
  Product4/1 -> Scope2/1, Display/1
  Gain/1 -> Product4/2
  l_DC_alfa/beta/2(Ibeta_sum) -> Terminator2/1  "I_beta_real"
  l_DC_alfa/beta/1(Ialfa_sum) -> Terminator1/1  "I_afa_real"
  Constant/1 -> Rotació/3(V_0_diff)
  Current Control/2(V_d_s) -> Conditional unit delay1/1  "V_0_s"
  [ids] -> Product3/2
  Product3/1 -> Sum1/1
  Sum3/1 -> Sum12/1
  scaling/1 -> Sum3/2
  [iqs] -> Product5/1
  Control Energies DC/1(Pt') -> Sum3/1
  Product5/1 -> Sum1/2
  Sum1/1 -> Gain6/1  "V_0_s"
  Gain6/1 -> scaling/1  "V_0_"
  [uq] -> Product5/2
  [ud] -> Product3/1
  Subsystem4/1(iqref) -> Current Control/1(Iq*)
  Is2/3(I_0_s) -> Terminator4/1  "I_0_s"
  Sum4/1 -> Conditional unit delay2/1
  Sum19/1 -> Control Energies DC/1(Pt)
  Sum12/1 -> Controladors/1(I_0_sum)
  Controladors/1(V_0_sum) -> Sum4/1
  [ud] -> Current Control/6(ud)
  [uq] -> Current Control/5(uq)
  Current Control/1(V_q_s) -> Conditional unit delay/1  "V_0_s"
  [angle] -> Rotació/4(Angle)
  [angle] -> Is/4(Angle)
  Calcul Energies2/2(Ebt) -> Sum18/2
  Calcul Energies2/3(Ect) -> Sum18/3
  Vs/1 -> Calcul Energies2/1(Vs)
  Iss/1 -> Demux/1
  Demux/3 -> [Ics]
  Demux/2 -> [Ibs]
  Demux/1 -> [Ias]
  Demux3/1 -> Is2/1(Ias)
  Demux3/3 -> Is2/3(Ics)
  U/1 -> Demux3/1
  PLL1/1(Angle) -> [angle]
  [angle] -> Is2/4(Angle)
  Demux3/2 -> Is2/2(Ibs)
  Demux1/2 -> [Ibu]
  Demux2/1 -> [Ial]
  Demux2/3 -> [Icl]
  Il/1 -> Demux2/1
  Demux1/3 -> [Icu]
  Demux1/1 -> [Iau]
  Demux2/2 -> [Ibl]
  Iu/1 -> Demux1/1
  Clarke Anti-Transformation2/3(Vc_sum) -> Mux/6  "Vcsum"
  Sum15/1 -> Product2/1
  [Icu] -> Sum15/2
  [Icl] -> Sum15/1
  Product2/1 -> Mux2/3  "Ic_sum"
  Sum14/1 -> Product1/1
  [Ibu] -> Sum14/2
  [Ibl] -> Sum14/1
  Product1/1 -> Mux2/2  "Ib_sum"
  Constant1/1 -> Product/2, Product1/2, Product2/2
  Sum13/1 -> Product/1
  [Iau] -> Sum13/2  "Iu"
  [Ial] -> Sum13/1  "Il"
  Product/1 -> Mux2/1  "Ia_sum"
  Mux2/1 -> l_DC_alfa/beta/1(Iabc_sum)
  Rotació/2(V_beta_diff) -> Clarke Anti-Transformation/2(V_beta_dfff)  "Vbeta_diffa"
  [Ibs] -> Is/2(Ibs)  "Ibs"
  [Ics] -> Is/3(Ics)  "Ics"
  [Ias] -> Is/1(Ias)  "Ias"
  Rotació/3(V_0) -> Clarke Anti-Transformation/3(V_0_diff)  "V_0_diff"
  Rotació/1(V_alfa_diff) -> Clarke Anti-Transformation/1(V_alfa_diff)  "Valfa_diff"
  Is/1(I_q_s) -> Conditional zoh/1  "I_q_s"
  Is/2(I_d_s) -> Conditional zoh1/1(In1)  "I_d_s"
  Clarke Anti-Transformation/1(Va_diff) -> Mux/1  "Vadiff"
  Clarke Anti-Transformation/2(Vb_diff) -> Mux/2  "Vbdiff"
  Clarke Anti-Transformation/3(Vc_diff) -> Mux/3  "Vcdiff"
  Clarke Anti-Transformation2/2(Vb_sum) -> Mux/5  "Vbsum"
  Clarke Anti-Transformation2/1(Va_sum) -> Mux/4  "Vasum"
  Mux/1 -> Vdiff-sum/1
  Constant3/1 -> Clarke Anti-Transformation2/2(V_beta_sum)
  Constant2/1 -> Clarke Anti-Transformation2/1(V_alfa_sum)
  Calcul Energies2/1(Eat) -> Sum18/1
  Ref Ptotal2/1 -> Sum19/2, Scope1/2  "Pref"
  Low-Pass Filter (Discrete or Continuous)/1 -> [iqs], Current Control/2(Iq)
  Low-Pass Filter (Discrete or Continuous)1/1 -> [ids], Current Control/4(Id)
  Low-Pass Filter (Discrete or Continuous)5/1 -> Conditional zoh6/1(In1)
  Low-Pass Filter (Discrete or Continuous)4/1 -> Conditional zoh5/1
  Low-Pass Filter (Discrete or Continuous)3/1 -> Conditional zoh4/1
  Low-Pass Filter (Discrete or Continuous)7/1 -> Conditional zoh2/1
  Is/3(I_0_s) -> Terminator/1
  Low-Pass Filter (Discrete or Continuous)6/1 -> Conditional zoh3/1
  Constant5/1 -> Subsystem4/2(vd_ref)
  Constant10/1 -> Subsystem4/1(vq_ref)
  [uq] -> Subsystem4/3(vq)
  [ud] -> Subsystem4/4(vd)
  Subsystem4/2(idref) -> Current Control/3(Id*)
  [uq] -> PLL1/3(uq)
  [ud] -> PLL1/5(ud)
  [iqs] -> PLL1/2(iqs)
  [ids] -> PLL1/4(ids)
  Constant4/1 -> PLL1/1(Pref)
  Conditional unit delay1/1 -> Rotació/2(V_d_diff)
  Conditional unit delay/1 -> Rotació/1(V_q_diff)
  Conditional zoh/1 -> Low-Pass Filter (Discrete or Continuous)/1
  Conditional zoh1/1(Out1) -> Low-Pass Filter (Discrete or Continuous)1/1
  Conditional unit delay2/1 -> Clarke Anti-Transformation2/3(V_0_sum)
  Vdc/1 -> Product4/1, Low-Pass Filter (Discrete or Continuous)7/1
  Conditional zoh2/1 -> Sum4/2
  Conditional zoh3/1 -> Sum12/2, To Workspace2/1, Display1/1, Gain/1
  l_DC_alfa/beta/3(I0_sum) -> Low-Pass Filter (Discrete or Continuous)6/1  "I_0_real"
  Is2/1(I_q_s) -> Low-Pass Filter (Discrete or Continuous)4/1
  Is2/2(I_d_s) -> Low-Pass Filter (Discrete or Continuous)5/1
  Conditional zoh6/1(Out1) -> [ud]
  Conditional zoh5/1 -> [uq]
  Sum18/1 -> Low-Pass Filter (Discrete or Continuous)3/1  "Preal"
  Conditional zoh4/1 -> Sum19/1

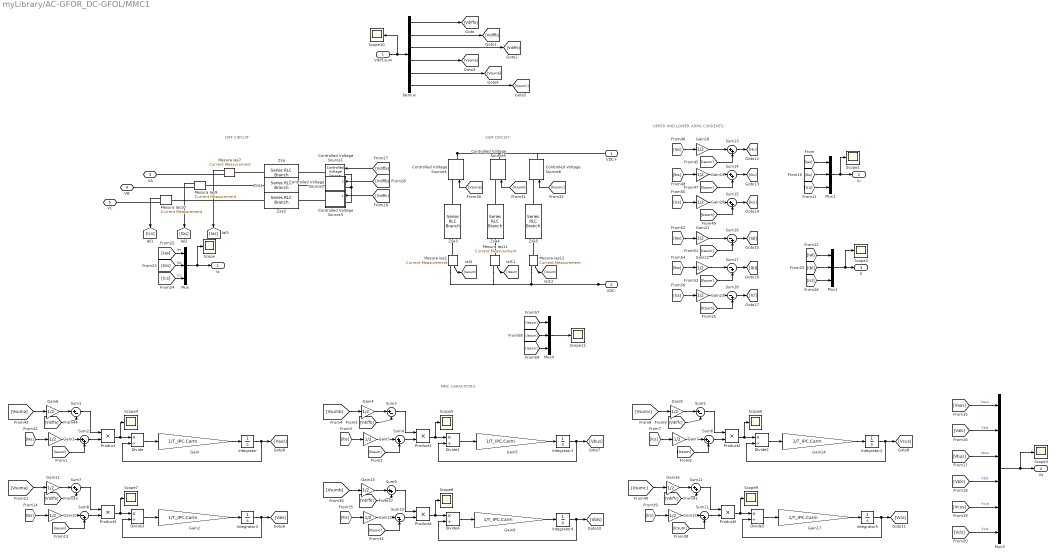
== system myLibrary/AC-GFOR_DC-GFOL/MMC1 ==
  note: UPPER AND LOWER ARMS CURRENTS:
  note: MMC CAPACITORS:
  note: SUM CIRCUIT:
  note: DIFF CIRCUIT:
  Vdiff,sum : Inport
  Controlled Voltage Source1 : spsControlledVoltageSourceLib/Controlled Voltage Source  Initialize=on  Source_Type=AC  Amplitude=initIPC.Udiff_mag  Phase=initIPC.angle_vdiff  Frequency=T_IPC.fb  Measurements=None
  Controlled Voltage Source2 : Subsystem  DialogController=POWERSYS.PowerSysDialog  LoadFcn=sps_rtmsupport('LoadFcn',gcbh);  StartFcn=sps_rtmsupport('StartFcn',gcbh);  StopFcn=sps_rtmsupport('StopFcn',gcbh);  mask(Controlled Voltage Source){Initialize=on, Source_Type=AC, Amplitude=initIPC.Udiff_mag, Phase=initIPC.angle_vdiff-120, Frequency=T_IPC.fb, Measurements=None}
      mask prompts: Source_Type "Source type"; Amplitude "Initial amplitude (V):"; Phase "Initial phase (deg):"; Frequency "Initial frequency (Hz):"
      mask help:
      | Converts the Simulink input signal into an equivalent voltage source. The generated voltage is driven by the input signal of the block.
      |
      | You can initialize your circuit with a specific AC or DC voltage. If you want to start the simulation in steady-state, the block input must be connected to a signal starting as a sinusoidal or DC waveform corresponding to the initial values.
      mask init:
      | powericon('psbloadfunction',gcb,'goto','Initialize');
      | powericon('ControlledSourcesCback',gcb);
      | power_initmask();
      settings: LibrarySourceBlock=spsControlledVoltageSourceLib/Controlled Voltage Source  CopyFcn=sps_rtmsupport('CopyFcn',gcbh); powericon('psbloadfunction',gcb,'goto','UpdateGotoTag');  DeleteFcn=sps_rtmsupport('DeleteFcn',gcbh);  UndoDeleteFcn=sps_rtmsupport('UndoDeleteFcn',gcbh);  ModelCloseFcn=sps_rtmsupport('ModelCloseFcn',gcbh);  PreSaveFcn=sps_rtmsupport('PreSaveFcn',gcbh);  PostSaveFcn=sps_rtmsupport('PostSaveFcn',gcbh);  NameChangeFcn=sps_rtmsupport('NameChangeFcn',gcbh);  PreCopyFcn=sps_rtmsupport('PreCopyFcn',gcbh);  OpenFcn=sps_rtmsupport('OpenFcn',gcbh, [1 2 6]);  CloseFcn=sps_rtmsupport('CloseFcn',gcbh);  PreDeleteFcn=sps_rtmsupport('PreDeleteFcn',gcbh);
      mask Help: helpview(psbhelp);
      mask Callback Initialize: powericon('ControlledSourcesCback',gcb);
      mask TypeOptions Source_Type: AC | DC
      mask Callback Source_Type: powericon('ControlledSourcesCback',gcb);
      mask TypeOptions Measurements: None | Voltage
      mask Display: plot(-50,-35,50,50-15,[0,9,18,24,29,30,29,24,18,9,0,-9,-18,-24,-29,-30,-29,-24,-18,-9,0],[30,29,24,18,9,0,-9,-18,-24,-29,-30,-29,-24,-18,-9,0,9,18,24,29,30],[0,9,18,24,29,30,29,24,18,9,0,-9,-18,-24,-29,-30,-29,-24,-18,-9,0]./-2.4,[1 2 3 4 5 6 7 8 9 10 11 12 13 14 15 16 17 18 19 20 21].*1.5-15);
  Controlled Voltage Source3 : Subsystem  DialogController=POWERSYS.PowerSysDialog  LoadFcn=sps_rtmsupport('LoadFcn',gcbh);  StartFcn=sps_rtmsupport('StartFcn',gcbh);  StopFcn=sps_rtmsupport('StopFcn',gcbh);  mask(Controlled Voltage Source){Initialize=on, Source_Type=AC, Amplitude=initIPC.Udiff_mag, Phase=initIPC.angle_vdiff+120, Frequency=T_IPC.fb, Measurements=None}
      mask prompts: Source_Type "Source type"; Amplitude "Initial amplitude (V):"; Phase "Initial phase (deg):"; Frequency "Initial frequency (Hz):"
      mask help:
      | Converts the Simulink input signal into an equivalent voltage source. The generated voltage is driven by the input signal of the block.
      |
      | You can initialize your circuit with a specific AC or DC voltage. If you want to start the simulation in steady-state, the block input must be connected to a signal starting as a sinusoidal or DC waveform corresponding to the initial values.
      mask init:
      | powericon('psbloadfunction',gcb,'goto','Initialize');
      | powericon('ControlledSourcesCback',gcb);
      | power_initmask();
      settings: LibrarySourceBlock=spsControlledVoltageSourceLib/Controlled Voltage Source  CopyFcn=sps_rtmsupport('CopyFcn',gcbh); powericon('psbloadfunction',gcb,'goto','UpdateGotoTag');  DeleteFcn=sps_rtmsupport('DeleteFcn',gcbh);  UndoDeleteFcn=sps_rtmsupport('UndoDeleteFcn',gcbh);  ModelCloseFcn=sps_rtmsupport('ModelCloseFcn',gcbh);  PreSaveFcn=sps_rtmsupport('PreSaveFcn',gcbh);  PostSaveFcn=sps_rtmsupport('PostSaveFcn',gcbh);  NameChangeFcn=sps_rtmsupport('NameChangeFcn',gcbh);  PreCopyFcn=sps_rtmsupport('PreCopyFcn',gcbh);  OpenFcn=sps_rtmsupport('OpenFcn',gcbh, [1 2 6]);  CloseFcn=sps_rtmsupport('CloseFcn',gcbh);  PreDeleteFcn=sps_rtmsupport('PreDeleteFcn',gcbh);
      mask Help: helpview(psbhelp);
      mask Callback Initialize: powericon('ControlledSourcesCback',gcb);
      mask TypeOptions Source_Type: AC | DC
      mask Callback Source_Type: powericon('ControlledSourcesCback',gcb);
      mask TypeOptions Measurements: None | Voltage
      mask Display: plot(-50,-35,50,50-15,[0,9,18,24,29,30,29,24,18,9,0,-9,-18,-24,-29,-30,-29,-24,-18,-9,0],[30,29,24,18,9,0,-9,-18,-24,-29,-30,-29,-24,-18,-9,0,9,18,24,29,30],[0,9,18,24,29,30,29,24,18,9,0,-9,-18,-24,-29,-30,-29,-24,-18,-9,0]./-2.4,[1 2 3 4 5 6 7 8 9 10 11 12 13 14 15 16 17 18 19 20 21].*1.5-15);
  Controlled Voltage Source4 : spsControlledVoltageSourceLib/Controlled Voltage Source  Initialize=on  Source_Type=DC  Amplitude=initIPC.Usuma  Phase=0  Frequency=0  Measurements=None
  Controlled Voltage Source5 : spsControlledVoltageSourceLib/Controlled Voltage Source  Initialize=on  Source_Type=DC  Amplitude=initIPC.Usumb  Phase=angle(Udiff_a)*180/pi  Frequency=60  Measurements=None
  Controlled Voltage Source6 : spsControlledVoltageSourceLib/Controlled Voltage Source  Initialize=on  Source_Type=DC  Amplitude=initIPC.Usumc  Phase=angle(Udiff_a)*180/pi  Frequency=60  Measurements=None
  Demux : Demux  Outputs=6
  Divide{,1..5} (6 alike) : Product  Inputs=*/
  Gain{,2,5,9,14,17} (6 alike) : Gain  Gain=1/T_IPC.Carm
  Gain{1,3..4,6..8,10..13,15..16,18..23} (18 alike) : Gain  Gain=1/2
  Integrator{,1..5} (6 alike) : Integrator  InitialCondition=1
  Mesura Ias{1,7,9..12} (6 alike) : spsCurrentMeasurementLib/Current Measurement  PhasorSimulation=off  OutputType=Complex  PSBequivalent=0
  Mux{,1..2,4} (4 alike) : Mux  Inputs=3
  Mux3 : Mux  Inputs=6
  Product{,1..5} (6 alike) : Product
  Scope{,1..11} (12 alike) : Scope
  Sum1 : Sum  Inputs=|+-
  Sum{8,10..11,16..18} (6 alike) : Sum  Inputs=|-+
  Sum{2,4,6..7,9,12..15} (9 alike) : Sum  Inputs=|++
  Sum3 : Sum  Inputs=|+-
  Sum5 : Sum  Inputs=|+-
  Zsa : spsSeriesRLCBranchLib/Series RLC Branch  LConnTagsString=__new0  RConnTagsString=__new0  BranchType=RL  Resistance=T_IPC.Rc+T_IPC.Ra/2  Inductance=T_IPC.Lc+T_IPC.La/2  SetiL0=on  InitialCurrent=initIPC.Isa  Capacitance=1e-6  Setx0=off  InitialVoltage=0  Measurements=None
  Zsa1 : spsSeriesRLCBranchLib/Series RLC Branch  LConnTagsString=__new0  RConnTagsString=__new0  BranchType=RL  Resistance=T_IPC.Rc+T_IPC.Ra/2  Inductance=T_IPC.Lc+T_IPC.La/2  SetiL0=on  InitialCurrent=initIPC.Isb  Capacitance=1e-6  Setx0=off  InitialVoltage=0  Measurements=None
  Zsa2 : spsSeriesRLCBranchLib/Series RLC Branch  LConnTagsString=__new0  RConnTagsString=__new0  BranchType=RL  Resistance=T_IPC.Rc+T_IPC.Ra/2  Inductance=T_IPC.Lc+T_IPC.La/2  SetiL0=on  InitialCurrent=initIPC.Isc  Capacitance=1e-6  Setx0=off  InitialVoltage=0  Measurements=None
  Zsa3 : spsSeriesRLCBranchLib/Series RLC Branch  LConnTagsString=__new0  RConnTagsString=__new0  BranchType=RL  Resistance=2*T_IPC.Ra  Inductance=2*T_IPC.La  SetiL0=on  InitialCurrent=initIPC.isum0_DC  Capacitance=1e-6  Setx0=off  InitialVoltage=0  Measurements=None
  Zsa4 : spsSeriesRLCBranchLib/Series RLC Branch  LConnTagsString=__new0  RConnTagsString=__new0  BranchType=RL  Resistance=2*T_IPC.Ra  Inductance=2*T_IPC.La  SetiL0=on  InitialCurrent=initIPC.isum0_DC  Capacitance=1e-6  Setx0=off  InitialVoltage=0  Measurements=None
  Zsa5 : spsSeriesRLCBranchLib/Series RLC Branch  LConnTagsString=__new0  RConnTagsString=__new0  BranchType=RL  Resistance=2*T_IPC.Ra  Inductance=2*T_IPC.La  SetiL0=on  InitialCurrent=initIPC.isum0_DC  Capacitance=1e-6  Setx0=off  InitialVoltage=0  Measurements=None
  VDC+ : PMIOPort  Side=Right
  VDC- : PMIOPort  Port=2  Side=Right
  VA : PMIOPort  Port=3  Side=Left
  VB : PMIOPort  Port=4  Side=Left
  VC : PMIOPort  Port=5  Side=Left
  Is : Outport
  Iu : Outport  Port=2
  Il : Outport  Port=3
  Vs : Outport  Port=4
  wires:
  [Ibl] -> Mux2/2
  Sum18/1 -> [Icl]
  Gain23/1 -> Sum18/1
  [Ics] -> Gain23/1
  [Icsum] -> Sum18/2
  [Ibsum] -> Sum17/2
  [Ibs] -> Gain22/1
  Gain22/1 -> Sum17/1
  Sum17/1 -> [Ibl]
  Sum16/1 -> [Ial]
  Gain21/1 -> Sum16/1
  [Ias] -> Gain21/1
  [Iasum] -> Sum16/2
  Sum15/1 -> [Icu]
  [Icsum] -> Sum15/2
  Gain20/1 -> Sum15/1
  [Ics] -> Gain20/1
  [Ibs] -> Gain19/1
  Gain19/1 -> Sum14/1
  [Ibsum] -> Sum14/2
  Sum14/1 -> [Ibu]
  Sum13/1 -> [Iau]
  [Iasum] -> Sum13/2
  Gain18/1 -> Sum13/1
  [Ias] -> Gain18/1
  Sum11/1 -> Product5/2
  Product5/1 -> Scope9/1, Divide5/1
  Divide5/1 -> Gain17/1
  Gain17/1 -> Integrator5/1
  Integrator5/1 -> [Vcls], Divide5/2
  Gain16/1 -> Sum12/1
  [Vdiffc] -> Sum12/2
  [Icsum] -> Sum11/2
  Gain15/1 -> Sum11/1
  [Ics] -> Gain15/1
  [Vsumc] -> Gain16/1
  Sum12/1 -> Product5/1
  Sum9/1 -> Product4/1
  [Vsumb] -> Gain13/1
  [Ibs] -> Gain12/1
  Gain12/1 -> Sum10/1
  [Ibsum] -> Sum10/2
  [Vdiffb] -> Sum9/2
  Gain13/1 -> Sum9/1
  Integrator4/1 -> Divide4/2, [Vbls]
  Gain9/1 -> Integrator4/1
  Divide4/1 -> Gain9/1
  Product4/1 -> Divide4/1, Scope8/1
  Sum10/1 -> Product4/2
  Sum8/1 -> Product3/2
  Product3/1 -> Scope7/1, Divide3/1
  Divide3/1 -> Gain2/1
  Gain2/1 -> Integrator3/1
  Integrator3/1 -> [Vals], Divide3/2
  Gain11/1 -> Sum7/1
  [Vdiffa] -> Sum7/2
  [Iasum] -> Sum8/2
  Gain10/1 -> Sum8/1
  [Ias] -> Gain10/1
  [Vsuma] -> Gain11/1
  Sum7/1 -> Product3/1
  Sum5/1 -> Product2/1
  [Vsumc] -> Gain8/1
  [Ics] -> Gain7/1
  Gain7/1 -> Sum6/1
  [Icsum] -> Sum6/2
  [Vdiffc] -> Sum5/2
  Gain8/1 -> Sum5/1
  Integrator2/1 -> Divide2/2, [Vcus]
  Gain14/1 -> Integrator2/1
  Divide2/1 -> Gain14/1
  Product2/1 -> Divide2/1, Scope6/1
  Sum6/1 -> Product2/2
  Sum4/1 -> Product1/2
  Product1/1 -> Scope5/1, Divide1/1
  Divide1/1 -> Gain5/1
  Gain5/1 -> Integrator1/1
  Integrator1/1 -> [Vbus], Divide1/2
  Gain4/1 -> Sum3/1
  [Vdiffb] -> Sum3/2
  [Ibsum] -> Sum4/2
  Gain3/1 -> Sum4/1
  [Ibs] -> Gain3/1
  [Vsumb] -> Gain4/1
  Sum3/1 -> Product1/1
  Sum1/1 -> Product/1
  [Vsuma] -> Gain6/1
  [Ias] -> Gain1/1
  Gain1/1 -> Sum2/1
  [Iasum] -> Sum2/2
  [Vdiffa] -> Sum1/2
  Gain6/1 -> Sum1/1
  [Vsumc] -> Controlled Voltage Source6/1
  [Vsumb] -> Controlled Voltage Source5/1
  [Vsuma] -> Controlled Voltage Source4/1
  Mesura Ias12/1 -> [Icsum]
  Mesura Ias11/1 -> [Ibsum]
  Mesura Ias1/1 -> [Iasum]
  [Vdiffc] -> Controlled Voltage Source3/1(s)
  [Vdiffb] -> Controlled Voltage Source2/1(s)
  [Vdiffa] -> Controlled Voltage Source1/1
  Integrator/1 -> Divide/2, [Vaus]
  Gain/1 -> Integrator/1
  Divide/1 -> Gain/1
  Product/1 -> Divide/1, Scope4/1
  Sum2/1 -> Product/2
  Mux3/1 -> Vs/1, Scope3/1
  [Vcls] -> Mux3/6  "Vcls"
  [Vcus] -> Mux3/5  "Vcus"
  [Vbls] -> Mux3/4  "Vbls"
  [Vbus] -> Mux3/3  "Vbus"
  [Vals] -> Mux3/2  "Vals"
  [Vaus] -> Mux3/1  "Vaus"
  [Icl] -> Mux2/3
  Mux2/1 -> Il/1, Scope2/1
  [Ial] -> Mux2/1
  Mux1/1 -> Iu/1, Scope1/1
  [Icu] -> Mux1/3
  [Ibu] -> Mux1/2
  [Iau] -> Mux1/1
  [Ias] -> Mux/1  "Ias"
  [Ibs] -> Mux/2  "Ibs"
  [Ics] -> Mux/3  "Ics"
  Mux/1 -> Is/1, Scope/1
  Demux/4 -> [Vsuma]
  Demux/2 -> [Vdiffb]
  Demux/3 -> [Vdiffc]
  Demux/1 -> [Vdiffa]
  Demux/6 -> [Vsumc]
  Demux/5 -> [Vsumb]
  Vdiff,sum/1 -> Scope10/1, Demux/1
  Mesura Ias9/1 -> [Ibs]
  Mesura Ias7/1 -> [Ias]
  Mesura Ias10/1 -> [Ics]
  [Iasum] -> Mux4/1
  [Iasum] -> Mux4/2
  [Iasum] -> Mux4/3
  Mux4/1 -> Scope11/1
  connections:
  VDC-/RConn1 -- Mesura Ias12/RConn1 -- Mesura Ias11/RConn1 -- Mesura Ias1/RConn1
  Controlled Voltage Source4/RConn1 -- Controlled Voltage Source5/RConn1 -- Controlled Voltage Source6/RConn1 -- VDC+/RConn1
  Controlled Voltage Source2/LConn1 -- Controlled Voltage Source3/LConn1 -- Controlled Voltage Source1/LConn1
  Controlled Voltage Source3/RConn1 -- Zsa2/LConn1
  Controlled Voltage Source2/RConn1 -- Zsa1/LConn1
  Controlled Voltage Source1/RConn1 -- Zsa/LConn1
  Zsa2/RConn1 -- Mesura Ias10/LConn1
  Zsa1/RConn1 -- Mesura Ias9/LConn1
  Zsa/RConn1 -- Mesura Ias7/LConn1
  Mesura Ias10/RConn1 -- VC/RConn1
  Mesura Ias9/RConn1 -- VB/RConn1
  Mesura Ias7/RConn1 -- VA/RConn1
  Zsa3/LConn1 -- Controlled Voltage Source4/LConn1
  Zsa3/RConn1 -- Mesura Ias1/LConn1
  Zsa4/LConn1 -- Controlled Voltage Source5/LConn1
  Zsa4/RConn1 -- Mesura Ias11/LConn1
  Zsa5/LConn1 -- Controlled Voltage Source6/LConn1
  Zsa5/RConn1 -- Mesura Ias12/LConn1
